simulink model "Proj2_P4_2"  (Simulink 8.6)
settings: Solver=ode45  StartTime=0.0  StopTime=10  MaxStep=0.001  RelTol=1e-3
values from neighbouring files (symbols this model uses):
  fl_rd_0 = fl_rd_rated    [Proj2_IM_IC_rated.m]    (also in Proj2_P1_calc.m = eps)
  fl_rd_0_est2 = fl_rd_rated_est2    [Proj2_P4_S2.m]    (also in Proj2_P4_calc2.m = fl_rd_0; Proj2_P4_calc3.m = fl_rd_0)
  fl_rd_0_est3 = fl_rd_rated    [Proj2_P4_S3.m]    (also in Proj2_P4_calc2.m = fl_rd_0; Proj2_P4_calc3.m = fl_rd_0)
  fl_sd_0 = fl_sd_rated    [Proj2_IM_IC_rated.m]    (also in Proj2_P1_calc.m = 0)
  fl_sq_0 = fl_sq_rated    [Proj2_IM_IC_rated.m]    (also in Proj2_P1_calc.m = 0)
  Isd_rated = real(Is_rated)    [Proj2_IM_IC_rated.m]
  Isd_rated_est2 = real(Is_rated_est2)    [Proj2_P4_S2.m]    (also in Proj2_P4_calc2.m = Isd_rated)
  Isd_rated_est3 = real(Is_rated_est3)    [Proj2_P4_S3.m]    (also in Proj2_P4_calc2.m = Isd_rated)
  Isq_0 = Isq_rated    [Proj2_IM_IC_rated.m]
  Isq_0_est2 = Isq_rated_est2    [Proj2_P4_S2.m]    (also in Proj2_P4_calc2.m = Isq_0; Proj2_P4_calc3.m = Isq_0)
  Isq_0_est3 = Isq_rated_est3    [Proj2_P4_S3.m]    (also in Proj2_P4_calc2.m = Isq_0; Proj2_P4_calc3.m = Isq_0)
  J_eq = 75    [Proj2_IM_parameters.m]
  Ki_i = w_c_i*sqrt(R_s^2+(w_c_i*L_s*sigma)^2) / sqrt(1+wc_Kp_by_Ki_for_i^2)    [Proj2_IM_IC_rated.m]
  Ki_i_est3 = w_c_i*sqrt(R_s^2+(w_c_i*L_s*sigma_est3)^2) / sqrt(1+wc_Kp_by_Ki_for_i_est3^2)    [Proj2_P4_S3.m]    (also in Proj2_P4_calc2.m = Ki_i)
  Ki_s = w_c_s^2*J_eq/(k*sqrt(1+tan(PM_s)^2))    [Proj2_IM_IC_rated.m]
  Ki_s_est2 = w_c_s^2*J_eq/(k_est2*sqrt(1+tan(PM_s)^2))    [Proj2_P4_S2.m]    (also in Proj2_P4_calc2.m = Ki_s)
  Ki_s_est3 = w_c_s^2*J_eq/(k_est3*sqrt(1+tan(PM_s)^2))    [Proj2_P4_S3.m]    (also in Proj2_P4_calc2.m = Ki_s)
  Kp_i = Ki_i * wc_Kp_by_Ki_for_i / w_c_i    [Proj2_IM_IC_rated.m]
  Kp_i_est3 = Ki_i_est3 * wc_Kp_by_Ki_for_i_est3 / w_c_i    [Proj2_P4_S3.m]    (also in Proj2_P4_calc2.m = Kp_i)
  Kp_s = Ki_s * wc_Kp_by_Ki_for_s / w_c_s    [Proj2_IM_IC_rated.m]
  Kp_s_est2 = Ki_s_est2 * wc_Kp_by_Ki_for_s / w_c_s    [Proj2_P4_S2.m]    (also in Proj2_P4_calc2.m = Kp_s)
  Kp_s_est3 = Ki_s_est3 * wc_Kp_by_Ki_for_s / w_c_s    [Proj2_P4_S3.m]    (also in Proj2_P4_calc2.m = Kp_s)
  L_m = X_m /w_syn    (= 0.00152788745368)    [Proj2_IM_parameters.m]
  L_r = L_lr+L_m    (= 0.00161011750761)    [Proj2_IM_parameters.m]
  L_r_est3 = L_lr_est3 + L_m    [Proj2_P4_S3.m]
  L_s = L_ls+L_m    (= 0.00161807525477)    [Proj2_IM_parameters.m]
  p = 6    [Proj2_IM_parameters.m]
  R_s = 1.4*10^-3    (= 0.0014)    [Proj2_IM_parameters.m]
  T_L_rated = T_em_rated    [Proj2_IM_parameters.m]
  tau_r = L_r/R_r    (= 1.62474016914)    [Proj2_IM_parameters.m]
  tau_r_est2 = L_r/R_r_est2    [Proj2_P4_S2.m]
  tau_r_est3 = L_r_est3/R_r    [Proj2_P4_S3.m]
  theta_da_0 = theta_fl_rated_a    [Proj2_IM_IC_rated.m]    (also in Proj2_P1_calc.m = 0)
  theta_dA_0 = theta_fl_rated_a    [Proj2_IM_IC_rated.m]    (also in Proj2_P1_calc.m = 0)
  theta_da_0_est2 = theta_fl_rated_a_est2    [Proj2_P4_S2.m]    (also in Proj2_P4_calc2.m = theta_da_0; Proj2_P4_calc3.m = theta_da_0)
  theta_da_0_est3 = theta_fl_rated_a_est3    [Proj2_P4_S3.m]    (also in Proj2_P4_calc2.m = theta_da_0; Proj2_P4_calc3.m = theta_da_0)
  Vsd_0 = Vsd_rated    [Proj2_IM_IC_rated.m]
  Vsd_prime_0 = Vsd_0 - L_m/L_r*d_fl_rd_0_by_dt + w_syn*sigma*L_s*Isq_0    [Proj2_IM_IC_rated.m]
  Vsq_0 = Vsq_rated    [Proj2_IM_IC_rated.m]
  Vsq_prime_0 = Vsq_0 - w_syn*(L_m/L_r)*fl_rd_0 - w_syn*sigma*L_s*Isd_0    [Proj2_IM_IC_rated.m]
  w_mech_0 = w_mech_rated    [Proj2_IM_IC_rated.m]    (also in Proj2_P1_calc.m = 0)
  w_mech_rated = (1-s)*w_syn/(p/2)    (= 124.407069082)    [Proj2_IM_parameters.m]
(part 1 of 2)
settings Model: Creator=XP  LastModifiedBy=XP
settings DataIOCC: SaveFormat=Dataset  SignalLoggingSaveFormat=Dataset
settings OptimizationCC: ExpressionDepthLimit=128
settings DebuggingCC: UnderspecifiedInitializationDetection=Simplified  MergeDetectMultiDrivingBlocksExec=error  SolverPrmCheckMsg=none  FcnCallInpInsideContextMsg=EnableAllAsError  StateNameClashWarn=none
settings HardwareCC: ProdBitPerPointer=64  ProdLargestAtomicFloat=Float  ProdIntDivRoundTo=Zero  ProdEndianess=LittleEndian  ProdWordSize=64  ProdHWDeviceType=Intel->x86-64 (Windows64)
settings GRTTargetCC: GeneratePreprocessorConditionals=Use local settings  CombineOutputUpdateFcns=on  GRTInterface=off
settings ConfigComp: CovModelRefEnable=off

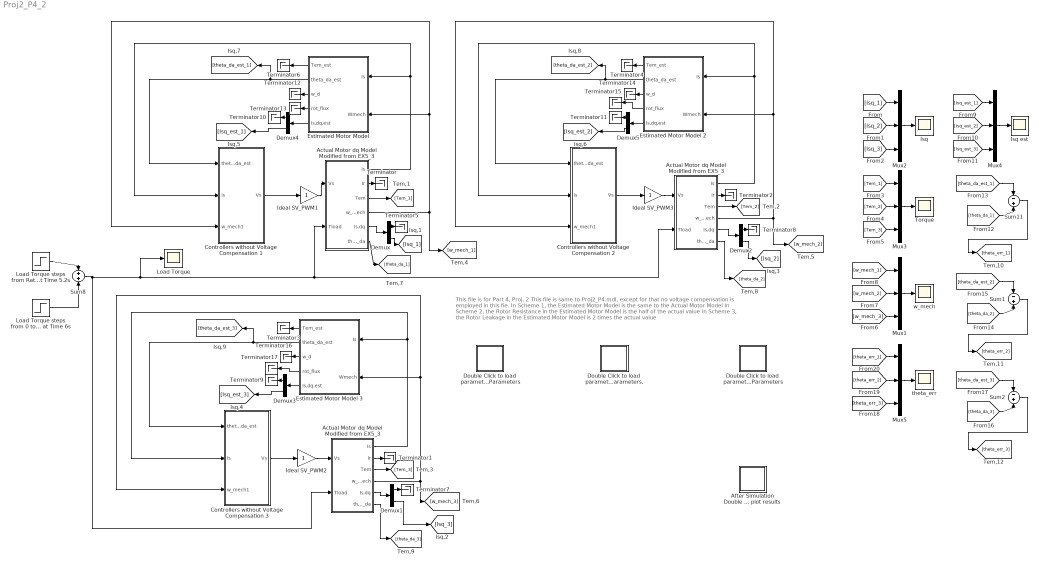
== system Proj2_P4_2 ==
  note: This file is for Part 4, Proj. 2
      | This file is same to Proj2_P4.mdl, except for that no voltage compensation is employed in this fie.
      |
      | In Scheme 1, the Estimated Motor Model is the same to the Actual Motor Model
      | In Scheme 2, the Rotor Resistance in the Estimated Motor Model is the half of the actual value
      | In Scheme 3, the Rotor Leakage in the Estimated Motor Model is 2 times the actual value
  Actual Motor dq Model Modified from EX5_3 : Subsystem
  "Actual Motor dq Model Modified from EX5_3 " : Subsystem
  "Actual Motor dq Model Modified from EX5_3  " : Subsystem
  "After Simulation Double Click to plot results " : Subsystem
      settings: OpenFcn=Proj2_P4_plots
      mask Display:
      | plot(0,0)
      | plot(100,100)
      | disp('Plot')
  Controllers without Voltage Compensation 1 : Subsystem
  Controllers without Voltage Compensation 2 : Subsystem
  Controllers without Voltage Compensation 3 : Subsystem
  Demux{,1..5} (6 alike) : Demux  Outputs=2
  "Double Click to load parameters and initial conditions  In this case, all initial values are obtained based on Actual Parameters;  parameters of Estimated Motor and Voltage Compensation Mode are based on Estimated Parameters;  paramters of  Controllers are based on Actual Parameters.  " : Subsystem
      settings: OpenFcn=Proj2_P4_calc2
      mask Display:
      | plot(0,0)
      | plot(100,100)
      | disp('Start')
  "Double Click to load parameters and initial conditions  In this case, all initial values are obtained based on Actual Parameters;  parameters of Estimated Motor and Voltage Compensation Model and Controllers are all based on Estimated Parameters  " : Subsystem
      settings: OpenFcn=Proj2_P4_calc3
      mask Display:
      | plot(0,0)
      | plot(100,100)
      | disp('Start')
  "Double Click to load parameters and initial conditions  In this case, all parameters and initial values in Estimated Motor, Voltage Compensation  and Controller Mode are based on Estimated Parameters" : Subsystem
      settings: OpenFcn=Proj2_P4_calc
      mask Display:
      | plot(0,0)
      | plot(100,100)
      | disp('Start')
  Estimated Motor Model : Subsystem
  Estimated Motor Model 2 : Subsystem
  Estimated Motor Model 3 : Subsystem
  Ideal SV_PWM1 : Gain  SaturateOnIntegerOverflow=on  OutDataTypeStr=Inherit: Same as input  ParamDataTypeStr=Inherit: Same as input
  Ideal SV_PWM2 : Gain  SaturateOnIntegerOverflow=on  OutDataTypeStr=Inherit: Same as input  ParamDataTypeStr=Inherit: Same as input
  Ideal SV_PWM3 : Gain  SaturateOnIntegerOverflow=on  OutDataTypeStr=Inherit: Same as input  ParamDataTypeStr=Inherit: Same as input
  Isq : Scope
  Isq est : Scope
  Load Torque : Scope
  Load Torque steps from 0 to 3/4Rated value at Time 6s : Step  Time=6  After=3/4*T_L_rated  SampleTime=0
  Load Torque steps from Rated to 0 at Time 5.2s : Step  Time=5.2  Before=T_L_rated  After=0  SampleTime=0
  Mux{1..5} (5 alike) : Mux  Inputs=3
  Sum1 : Sum  Inputs=-|+  SaturateOnIntegerOverflow=on  InputSameDT=on  OutDataTypeStr=Inherit: Same as first input
  Sum11 : Sum  Inputs=-|+  SaturateOnIntegerOverflow=on  InputSameDT=on  OutDataTypeStr=Inherit: Same as first input
  Sum2 : Sum  Inputs=-|+  SaturateOnIntegerOverflow=on  InputSameDT=on  OutDataTypeStr=Inherit: Same as first input
  Sum8 : Sum  SaturateOnIntegerOverflow=on  InputSameDT=on  OutDataTypeStr=Inherit: Same as first input
  Terminator{,1..17} (18 alike) : Terminator
  Torque : Scope
  theta_err : Scope
  w_mech : Scope
  wires:
  Actual Motor dq Model Modified from EX5_3/2(Ir) -> Terminator/1
  Ideal SV_PWM1/1 -> Actual Motor dq Model Modified from EX5_3/1(Vs)
  Actual Motor dq Model Modified from EX5_3/1(Is) -> Controllers without Voltage Compensation 1/2(Is), Estimated Motor Model/1(Is)
  Controllers without Voltage Compensation 1/1(Vs) -> Ideal SV_PWM1/1
  Estimated Motor Model/2(theta_da_est) -> [theta_da_est_1], Controllers without Voltage Compensation 1/1(theta_da_est)
  Actual Motor dq Model Modified from EX5_3/4(w_mech) -> [w_mech_1], Controllers without Voltage Compensation 1/3(w_mech1), Estimated Motor Model/2(Wmech)
  "Actual Motor dq Model Modified from EX5_3  "/2(Ir) -> Terminator1/1
  Ideal SV_PWM2/1 -> "Actual Motor dq Model Modified from EX5_3  "/1(Vs)
  "Actual Motor dq Model Modified from EX5_3  "/1(Is) -> Controllers without Voltage Compensation 3/2(Is), Estimated Motor Model 3/1(Is)
  Estimated Motor Model 3/2(theta_da_est) -> [theta_da_est_3], Controllers without Voltage Compensation 3/1(theta_da_est)
  "Actual Motor dq Model Modified from EX5_3  "/4(w_mech) -> [w_mech_3], Controllers without Voltage Compensation 3/3(w_mech1), Estimated Motor Model 3/2(Wmech)
  "Actual Motor dq Model Modified from EX5_3 "/2(Ir) -> Terminator2/1
  Ideal SV_PWM3/1 -> "Actual Motor dq Model Modified from EX5_3 "/1(Vs)
  Sum8/1 -> "Actual Motor dq Model Modified from EX5_3  "/2(Tload), "Actual Motor dq Model Modified from EX5_3 "/2(Tload), Actual Motor dq Model Modified from EX5_3/2(Tload), Load Torque/1
  "Actual Motor dq Model Modified from EX5_3 "/1(Is) -> Estimated Motor Model 2/1(Is), Controllers without Voltage Compensation 2/2(Is)
  Estimated Motor Model 2/2(theta_da_est) -> [theta_da_est_2], Controllers without Voltage Compensation 2/1(theta_da_est)
  "Actual Motor dq Model Modified from EX5_3 "/4(w_mech) -> [w_mech_2], Controllers without Voltage Compensation 2/3(w_mech1), Estimated Motor Model 2/2(Wmech)
  Controllers without Voltage Compensation 3/1(Vs) -> Ideal SV_PWM2/1
  Controllers without Voltage Compensation 2/1(Vs) -> Ideal SV_PWM3/1
  Estimated Motor Model/1(Tem_est) -> Terminator6/1
  Estimated Motor Model 3/1(Tem_est) -> Terminator3/1
  Estimated Motor Model 2/1(Tem_est) -> Terminator4/1
  Actual Motor dq Model Modified from EX5_3/5(Is,dq) -> Demux/1
  Demux/1 -> Terminator5/1
  "Actual Motor dq Model Modified from EX5_3  "/5(Is,dq) -> Demux1/1
  Demux1/1 -> Terminator7/1
  "Actual Motor dq Model Modified from EX5_3 "/5(Is,dq) -> Demux2/1
  Demux2/1 -> Terminator8/1
  Demux/2 -> [Isq_1]
  Demux1/2 -> [Isq_3]
  Demux2/2 -> [Isq_2]
  Actual Motor dq Model Modified from EX5_3/3(Tem) -> [Tem_1]
  "Actual Motor dq Model Modified from EX5_3 "/3(Tem) -> [Tem_2]
  "Actual Motor dq Model Modified from EX5_3  "/3(Tem) -> [Tem_3]
  Estimated Motor Model 3/5(Is,dq,est) -> Demux3/1
  Demux3/1 -> Terminator9/1
  Demux3/2 -> [Isq_est_3]
  Estimated Motor Model/5(Is,dq,est) -> Demux4/1
  Demux4/1 -> Terminator10/1
  Demux4/2 -> [Isq_est_1]
  Estimated Motor Model 2/5(Is,dq,est) -> Demux5/1
  Demux5/1 -> Terminator11/1
  Demux5/2 -> [Isq_est_2]
  Actual Motor dq Model Modified from EX5_3/6(theta_da) -> [theta_da_1]
  "Actual Motor dq Model Modified from EX5_3 "/6(theta_da) -> [theta_da_2]
  "Actual Motor dq Model Modified from EX5_3  "/6(theta_da) -> [theta_da_3]
  Load Torque steps from Rated to 0 at Time 5.2s/1 -> Sum8/1
  Load Torque steps from 0 to 3/4Rated value at Time 6s/1 -> Sum8/2
  [theta_err_1] -> Mux5/1
  Mux3/1 -> Torque/1
  Mux1/1 -> w_mech/1
  [Tem_2] -> Mux3/2
  [Tem_3] -> Mux3/3
  [w_mech_3] -> Mux1/3
  [w_mech_2] -> Mux1/2
  [w_mech_1] -> Mux1/1
  [Isq_1] -> Mux2/1
  [Isq_2] -> Mux2/2
  [Isq_3] -> Mux2/3
  Mux2/1 -> Isq/1
  [Tem_1] -> Mux3/1
  [Isq_est_1] -> Mux4/1
  [Isq_est_2] -> Mux4/2
  [Isq_est_3] -> Mux4/3
  Mux4/1 -> Isq est/1
  [theta_da_est_1] -> Sum11/1
  [theta_da_1] -> Sum11/2
  [theta_da_est_2] -> Sum1/1
  [theta_da_2] -> Sum1/2
  [theta_da_est_3] -> Sum2/1
  [theta_da_3] -> Sum2/2
  Sum11/1 -> [theta_err_1]
  Sum1/1 -> [theta_err_2]
  Sum2/1 -> [theta_err_3]
  Mux5/1 -> theta_err/1
  [theta_err_3] -> Mux5/3
  [theta_err_2] -> Mux5/2
  Estimated Motor Model/3(w_d) -> Terminator12/1
  Estimated Motor Model/4(rot_flux) -> Terminator13/1
  Estimated Motor Model 2/3(w_d) -> Terminator14/1
  Estimated Motor Model 2/4(rot_flux) -> Terminator15/1
  Estimated Motor Model 3/3(w_d) -> Terminator16/1
  Estimated Motor Model 3/4(rot_flux) -> Terminator17/1

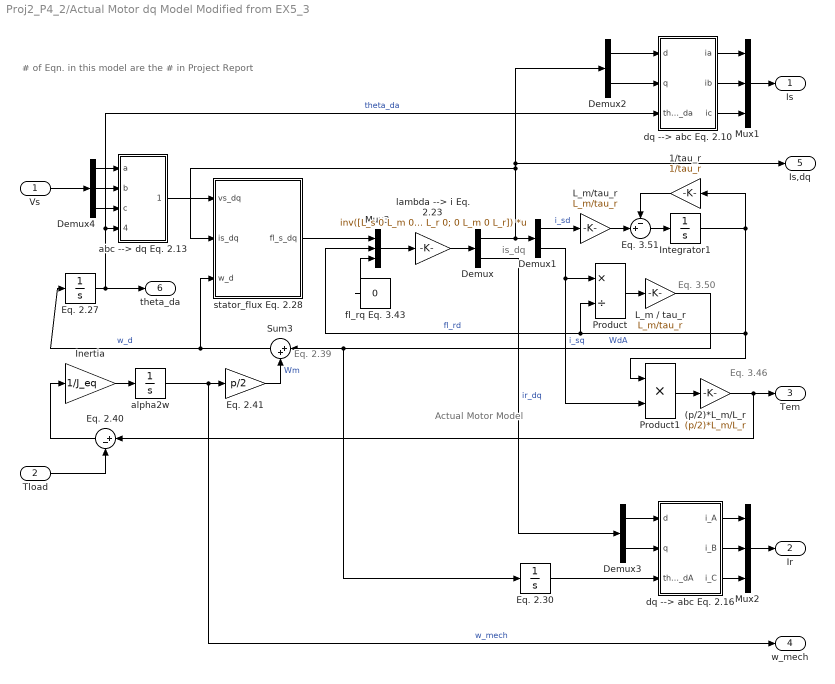
== system Proj2_P4_2/Actual Motor dq Model Modified from EX5_3 ==
  note: Eq. 2.39
  note: Eq. 3.46
  note: Eq. 3.50
  note: # of Eqn. in this model are the # in Project Report
  note: Actual Motor Model
  note: is_dq
  Vs : Inport
  Tload : Inport  Port=2
  (p/2)*L_m/L_r : Gain  Gain=(p/2)*L_m/L_r  SaturateOnIntegerOverflow=on  OutDataTypeStr=Inherit: Same as input  ParamDataTypeStr=Inherit: Same as input
  1/tau_r : Gain  Gain=1/tau_r  SaturateOnIntegerOverflow=on  OutDataTypeStr=Inherit: Same as input  ParamDataTypeStr=Inherit: Same as input
  Demux{,1..3} (4 alike) : Demux  Outputs=2
  Demux4 : Demux  Outputs=3
  Eq. 2.27 : Integrator  InitialCondition=theta_da_0
  Eq. 2.30 : Integrator  InitialCondition=theta_dA_0
  Eq. 2.40 : Sum  Inputs=|+-  SaturateOnIntegerOverflow=on  InputSameDT=on  OutDataTypeStr=Inherit: Same as first input
  Eq. 2.41 : Gain  Gain=p/2  SaturateOnIntegerOverflow=on  OutDataTypeStr=Inherit: Same as input  ParamDataTypeStr=Inherit: Same as input
  Eq. 3.51 : Sum  Inputs=-+|  SaturateOnIntegerOverflow=on  InputSameDT=on  OutDataTypeStr=Inherit: Same as first input
  Inertia : Gain  Gain=1/J_eq  SaturateOnIntegerOverflow=on  OutDataTypeStr=Inherit: Same as input  ParamDataTypeStr=Inherit: Same as input
  Integrator1 : Integrator  InitialCondition=fl_rd_0
  L_m / tau_r : Gain  Gain=L_m/tau_r  SaturateOnIntegerOverflow=on  OutDataTypeStr=Inherit: Same as input  ParamDataTypeStr=Inherit: Same as input
  L_m/tau_r : Gain  Gain=L_m/tau_r  SaturateOnIntegerOverflow=on  OutDataTypeStr=Inherit: Same as input  ParamDataTypeStr=Inherit: Same as input
  Mux1 : Mux  Inputs=3
  Mux2 : Mux  Inputs=3
  Mux3 : Mux  Inputs=3
  Product : Product  Inputs=*/  SaturateOnIntegerOverflow=on  RndMeth=Zero  InputSameDT=on  OutDataTypeStr=Inherit: Same as first input
  Product1 : Product  SaturateOnIntegerOverflow=on  RndMeth=Zero  InputSameDT=on  OutDataTypeStr=Inherit: Same as first input
  Sum3 : Sum  Inputs=|++  SaturateOnIntegerOverflow=on  InputSameDT=on  OutDataTypeStr=Inherit: Same as first input
  abc --> dq Eq. 2.13 : Subsystem
  alpha2w : Integrator  InitialCondition=w_mech_0
  dq --> abc Eq. 2.10 : Subsystem
  "dq --> abc Eq. 2.16 " : Subsystem
  fl_rq Eq. 3.43 : Constant  Value=0
  lambda --> i Eq. 2.23 : Gain  Gain=inv([L_s 0 L_m 0; 0 L_s 0 L_m; L_m 0 L_r 0; 0 L_m 0 L_r])  Multiplication=Matrix(K*u)  SaturateOnIntegerOverflow=on  OutDataTypeStr=Inherit: Same as input  ParamDataTypeStr=Inherit: Same as input
  stator_flux Eq. 2.28 : Subsystem
  Is : Outport
  Ir : Outport  Port=2
  Tem : Outport  Port=3
  w_mech : Outport  Port=4
  Is,dq : Outport  Port=5
  theta_da : Outport  Port=6
  wires:
  Mux3/1 -> lambda --> i Eq. 2.23/1
  Demux/1 -> Demux1/1, Is,dq/1, Demux2/1, stator_flux Eq. 2.28/2(is_dq)
  Eq. 2.27/1 -> theta_da/1, dq --> abc Eq. 2.10/3(theta_da), abc --> dq Eq. 2.13/4(theta_da)  "theta_da"
  stator_flux Eq. 2.28/1(fl_s_dq) -> Mux3/1
  abc --> dq Eq. 2.13/1(vs_dq) -> stator_flux Eq. 2.28/1(vs_dq)
  lambda --> i Eq. 2.23/1 -> Demux/1
  Demux1/1 -> L_m/tau_r/1  "i_sd"
  L_m/tau_r/1 -> Eq. 3.51/2
  1/tau_r/1 -> Eq. 3.51/1
  Eq. 3.51/1 -> Integrator1/1
  Demux1/2 -> Product/1, Product1/2  "i_sq"
  Product/1 -> L_m / tau_r/1
  L_m / tau_r/1 -> Sum3/1, Eq. 2.30/1  "WdA"
  Product1/1 -> (p/2)*L_m/L_r/1
  fl_rq Eq. 3.43/1 -> Mux3/3
  Sum3/1 -> Eq. 2.27/1, stator_flux Eq. 2.28/3(w_d)  "w_d"
  (p/2)*L_m/L_r/1 -> Tem/1, Eq. 2.40/1
  Demux2/1 -> dq --> abc Eq. 2.10/1(d)
  Demux2/2 -> dq --> abc Eq. 2.10/2(q)
  dq --> abc Eq. 2.10/1(ia) -> Mux1/1
  dq --> abc Eq. 2.10/2(ib) -> Mux1/2
  dq --> abc Eq. 2.10/3(ic) -> Mux1/3
  Integrator1/1 -> 1/tau_r/1, Mux3/2, Product/2, Product1/1  "fl_rd"
  Eq. 2.41/1 -> Sum3/2  "Wm"
  Demux/2 -> Demux3/1  "ir_dq"
  Eq. 2.40/1 -> Inertia/1
  Inertia/1 -> alpha2w/1
  alpha2w/1 -> w_mech/1, Eq. 2.41/1  "w_mech"
  Tload/1 -> Eq. 2.40/2
  Mux1/1 -> Is/1
  Demux3/1 -> "dq --> abc Eq. 2.16 "/1(d)
  Demux3/2 -> "dq --> abc Eq. 2.16 "/2(q)
  Eq. 2.30/1 -> "dq --> abc Eq. 2.16 "/3(theta_dA)
  "dq --> abc Eq. 2.16 "/1(i_A) -> Mux2/1
  "dq --> abc Eq. 2.16 "/2(i_B) -> Mux2/2
  "dq --> abc Eq. 2.16 "/3(i_C) -> Mux2/3
  Mux2/1 -> Ir/1
  Demux4/1 -> abc --> dq Eq. 2.13/1(a)
  Demux4/2 -> abc --> dq Eq. 2.13/2(b)
  Demux4/3 -> abc --> dq Eq. 2.13/3(c)
  Vs/1 -> Demux4/1

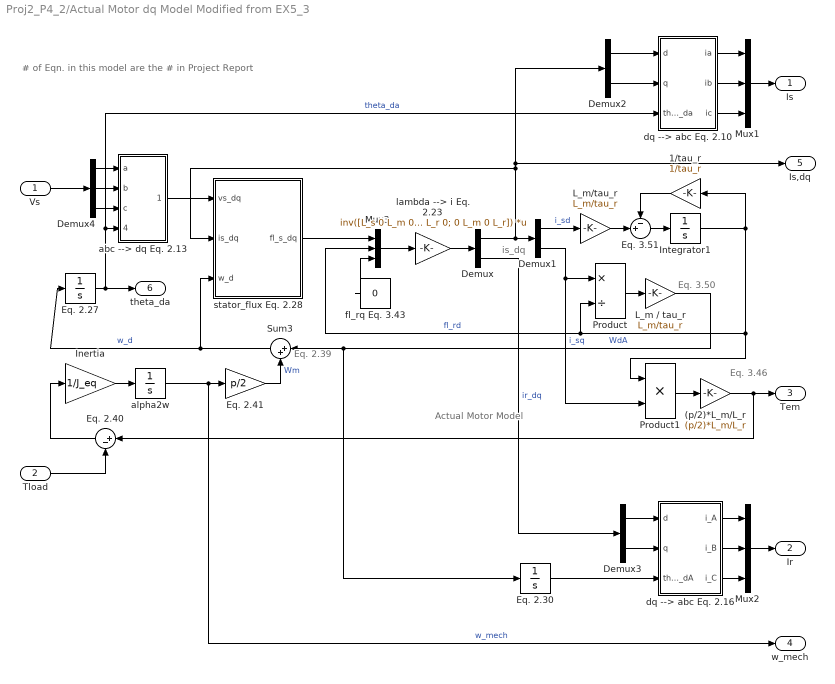
== system Proj2_P4_2/Actual Motor dq Model Modified from EX5_3  ==
  note: Eq. 2.39
  note: Eq. 3.46
  note: Eq. 3.50
  note: # of Eqn. in this model are the # in Project Report
  note: Actual Motor Model
  note: is_dq
  Vs : Inport
  Tload : Inport  Port=2
  (p/2)*L_m/L_r : Gain  Gain=(p/2)*L_m/L_r  SaturateOnIntegerOverflow=on  OutDataTypeStr=Inherit: Same as input  ParamDataTypeStr=Inherit: Same as input
  1/tau_r : Gain  Gain=1/tau_r  SaturateOnIntegerOverflow=on  OutDataTypeStr=Inherit: Same as input  ParamDataTypeStr=Inherit: Same as input
  Demux{,1..3} (4 alike) : Demux  Outputs=2
  Demux4 : Demux  Outputs=3
  Eq. 2.27 : Integrator  InitialCondition=theta_da_0
  Eq. 2.30 : Integrator  InitialCondition=theta_dA_0
  Eq. 2.40 : Sum  Inputs=|+-  SaturateOnIntegerOverflow=on  InputSameDT=on  OutDataTypeStr=Inherit: Same as first input
  Eq. 2.41 : Gain  Gain=p/2  SaturateOnIntegerOverflow=on  OutDataTypeStr=Inherit: Same as input  ParamDataTypeStr=Inherit: Same as input
  Eq. 3.51 : Sum  Inputs=-+|  SaturateOnIntegerOverflow=on  InputSameDT=on  OutDataTypeStr=Inherit: Same as first input
  Inertia : Gain  Gain=1/J_eq  SaturateOnIntegerOverflow=on  OutDataTypeStr=Inherit: Same as input  ParamDataTypeStr=Inherit: Same as input
  Integrator1 : Integrator  InitialCondition=fl_rd_0
  L_m / tau_r : Gain  Gain=L_m/tau_r  SaturateOnIntegerOverflow=on  OutDataTypeStr=Inherit: Same as input  ParamDataTypeStr=Inherit: Same as input
  L_m/tau_r : Gain  Gain=L_m/tau_r  SaturateOnIntegerOverflow=on  OutDataTypeStr=Inherit: Same as input  ParamDataTypeStr=Inherit: Same as input
  Mux1 : Mux  Inputs=3
  Mux2 : Mux  Inputs=3
  Mux3 : Mux  Inputs=3
  Product : Product  Inputs=*/  SaturateOnIntegerOverflow=on  RndMeth=Zero  InputSameDT=on  OutDataTypeStr=Inherit: Same as first input
  Product1 : Product  SaturateOnIntegerOverflow=on  RndMeth=Zero  InputSameDT=on  OutDataTypeStr=Inherit: Same as first input
  Sum3 : Sum  Inputs=|++  SaturateOnIntegerOverflow=on  InputSameDT=on  OutDataTypeStr=Inherit: Same as first input
  abc --> dq Eq. 2.13 : Subsystem
  alpha2w : Integrator  InitialCondition=w_mech_0
  dq --> abc Eq. 2.10 : Subsystem
  "dq --> abc Eq. 2.16 " : Subsystem
  fl_rq Eq. 3.43 : Constant  Value=0
  lambda --> i Eq. 2.23 : Gain  Gain=inv([L_s 0 L_m 0; 0 L_s 0 L_m; L_m 0 L_r 0; 0 L_m 0 L_r])  Multiplication=Matrix(K*u)  SaturateOnIntegerOverflow=on  OutDataTypeStr=Inherit: Same as input  ParamDataTypeStr=Inherit: Same as input
  stator_flux Eq. 2.28 : Subsystem
  Is : Outport
  Ir : Outport  Port=2
  Tem : Outport  Port=3
  w_mech : Outport  Port=4
  Is,dq : Outport  Port=5
  theta_da : Outport  Port=6
  wires:
  Mux3/1 -> lambda --> i Eq. 2.23/1
  Demux/1 -> Demux1/1, Is,dq/1, Demux2/1, stator_flux Eq. 2.28/2(is_dq)
  Eq. 2.27/1 -> theta_da/1, dq --> abc Eq. 2.10/3(theta_da), abc --> dq Eq. 2.13/4(theta_da)  "theta_da"
  stator_flux Eq. 2.28/1(fl_s_dq) -> Mux3/1
  abc --> dq Eq. 2.13/1(vs_dq) -> stator_flux Eq. 2.28/1(vs_dq)
  lambda --> i Eq. 2.23/1 -> Demux/1
  Demux1/1 -> L_m/tau_r/1  "i_sd"
  L_m/tau_r/1 -> Eq. 3.51/2
  1/tau_r/1 -> Eq. 3.51/1
  Eq. 3.51/1 -> Integrator1/1
  Demux1/2 -> Product/1, Product1/2  "i_sq"
  Product/1 -> L_m / tau_r/1
  L_m / tau_r/1 -> Sum3/1, Eq. 2.30/1  "WdA"
  Product1/1 -> (p/2)*L_m/L_r/1
  fl_rq Eq. 3.43/1 -> Mux3/3
  Sum3/1 -> Eq. 2.27/1, stator_flux Eq. 2.28/3(w_d)  "w_d"
  (p/2)*L_m/L_r/1 -> Tem/1, Eq. 2.40/1
  Demux2/1 -> dq --> abc Eq. 2.10/1(d)
  Demux2/2 -> dq --> abc Eq. 2.10/2(q)
  dq --> abc Eq. 2.10/1(ia) -> Mux1/1
  dq --> abc Eq. 2.10/2(ib) -> Mux1/2
  dq --> abc Eq. 2.10/3(ic) -> Mux1/3
  Integrator1/1 -> 1/tau_r/1, Mux3/2, Product/2, Product1/1  "fl_rd"
  Eq. 2.41/1 -> Sum3/2  "Wm"
  Demux/2 -> Demux3/1  "ir_dq"
  Eq. 2.40/1 -> Inertia/1
  Inertia/1 -> alpha2w/1
  alpha2w/1 -> w_mech/1, Eq. 2.41/1  "w_mech"
  Tload/1 -> Eq. 2.40/2
  Mux1/1 -> Is/1
  Demux3/1 -> "dq --> abc Eq. 2.16 "/1(d)
  Demux3/2 -> "dq --> abc Eq. 2.16 "/2(q)
  Eq. 2.30/1 -> "dq --> abc Eq. 2.16 "/3(theta_dA)
  "dq --> abc Eq. 2.16 "/1(i_A) -> Mux2/1
  "dq --> abc Eq. 2.16 "/2(i_B) -> Mux2/2
  "dq --> abc Eq. 2.16 "/3(i_C) -> Mux2/3
  Mux2/1 -> Ir/1
  Demux4/1 -> abc --> dq Eq. 2.13/1(a)
  Demux4/2 -> abc --> dq Eq. 2.13/2(b)
  Demux4/3 -> abc --> dq Eq. 2.13/3(c)
  Vs/1 -> Demux4/1

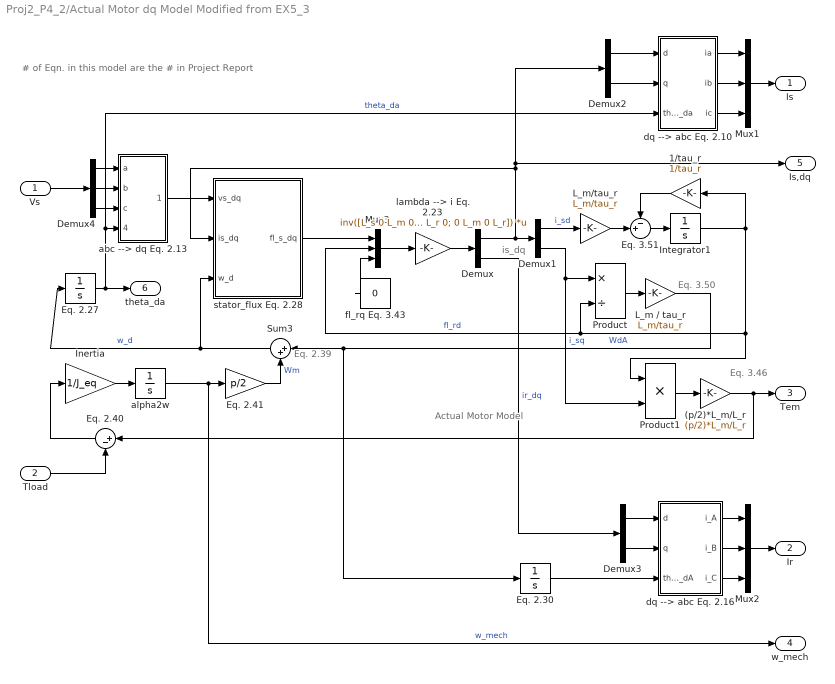
== system Proj2_P4_2/Actual Motor dq Model Modified from EX5_3   ==
  note: Eq. 2.39
  note: Eq. 3.46
  note: Eq. 3.50
  note: # of Eqn. in this model are the # in Project Report
  note: Actual Motor Model
  note: is_dq
  Vs : Inport
  Tload : Inport  Port=2
  (p/2)*L_m/L_r : Gain  Gain=(p/2)*L_m/L_r  SaturateOnIntegerOverflow=on  OutDataTypeStr=Inherit: Same as input  ParamDataTypeStr=Inherit: Same as input
  1/tau_r : Gain  Gain=1/tau_r  SaturateOnIntegerOverflow=on  OutDataTypeStr=Inherit: Same as input  ParamDataTypeStr=Inherit: Same as input
  Demux{,1..3} (4 alike) : Demux  Outputs=2
  Demux4 : Demux  Outputs=3
  Eq. 2.27 : Integrator  InitialCondition=theta_da_0
  Eq. 2.30 : Integrator  InitialCondition=theta_dA_0
  Eq. 2.40 : Sum  Inputs=|+-  SaturateOnIntegerOverflow=on  InputSameDT=on  OutDataTypeStr=Inherit: Same as first input
  Eq. 2.41 : Gain  Gain=p/2  SaturateOnIntegerOverflow=on  OutDataTypeStr=Inherit: Same as input  ParamDataTypeStr=Inherit: Same as input
  Eq. 3.51 : Sum  Inputs=-+|  SaturateOnIntegerOverflow=on  InputSameDT=on  OutDataTypeStr=Inherit: Same as first input
  Inertia : Gain  Gain=1/J_eq  SaturateOnIntegerOverflow=on  OutDataTypeStr=Inherit: Same as input  ParamDataTypeStr=Inherit: Same as input
  Integrator1 : Integrator  InitialCondition=fl_rd_0
  L_m / tau_r : Gain  Gain=L_m/tau_r  SaturateOnIntegerOverflow=on  OutDataTypeStr=Inherit: Same as input  ParamDataTypeStr=Inherit: Same as input
  L_m/tau_r : Gain  Gain=L_m/tau_r  SaturateOnIntegerOverflow=on  OutDataTypeStr=Inherit: Same as input  ParamDataTypeStr=Inherit: Same as input
  Mux1 : Mux  Inputs=3
  Mux2 : Mux  Inputs=3
  Mux3 : Mux  Inputs=3
  Product : Product  Inputs=*/  SaturateOnIntegerOverflow=on  RndMeth=Zero  InputSameDT=on  OutDataTypeStr=Inherit: Same as first input
  Product1 : Product  SaturateOnIntegerOverflow=on  RndMeth=Zero  InputSameDT=on  OutDataTypeStr=Inherit: Same as first input
  Sum3 : Sum  Inputs=|++  SaturateOnIntegerOverflow=on  InputSameDT=on  OutDataTypeStr=Inherit: Same as first input
  abc --> dq Eq. 2.13 : Subsystem
  alpha2w : Integrator  InitialCondition=w_mech_0
  dq --> abc Eq. 2.10 : Subsystem
  "dq --> abc Eq. 2.16 " : Subsystem
  fl_rq Eq. 3.43 : Constant  Value=0
  lambda --> i Eq. 2.23 : Gain  Gain=inv([L_s 0 L_m 0; 0 L_s 0 L_m; L_m 0 L_r 0; 0 L_m 0 L_r])  Multiplication=Matrix(K*u)  SaturateOnIntegerOverflow=on  OutDataTypeStr=Inherit: Same as input  ParamDataTypeStr=Inherit: Same as input
  stator_flux Eq. 2.28 : Subsystem
  Is : Outport
  Ir : Outport  Port=2
  Tem : Outport  Port=3
  w_mech : Outport  Port=4
  Is,dq : Outport  Port=5
  theta_da : Outport  Port=6
  wires:
  Mux3/1 -> lambda --> i Eq. 2.23/1
  Demux/1 -> Demux1/1, Is,dq/1, Demux2/1, stator_flux Eq. 2.28/2(is_dq)
  Eq. 2.27/1 -> theta_da/1, dq --> abc Eq. 2.10/3(theta_da), abc --> dq Eq. 2.13/4(theta_da)  "theta_da"
  stator_flux Eq. 2.28/1(fl_s_dq) -> Mux3/1
  abc --> dq Eq. 2.13/1(vs_dq) -> stator_flux Eq. 2.28/1(vs_dq)
  lambda --> i Eq. 2.23/1 -> Demux/1
  Demux1/1 -> L_m/tau_r/1  "i_sd"
  L_m/tau_r/1 -> Eq. 3.51/2
  1/tau_r/1 -> Eq. 3.51/1
  Eq. 3.51/1 -> Integrator1/1
  Demux1/2 -> Product/1, Product1/2  "i_sq"
  Product/1 -> L_m / tau_r/1
  L_m / tau_r/1 -> Sum3/1, Eq. 2.30/1  "WdA"
  Product1/1 -> (p/2)*L_m/L_r/1
  fl_rq Eq. 3.43/1 -> Mux3/3
  Sum3/1 -> Eq. 2.27/1, stator_flux Eq. 2.28/3(w_d)  "w_d"
  (p/2)*L_m/L_r/1 -> Tem/1, Eq. 2.40/1
  Demux2/1 -> dq --> abc Eq. 2.10/1(d)
  Demux2/2 -> dq --> abc Eq. 2.10/2(q)
  dq --> abc Eq. 2.10/1(ia) -> Mux1/1
  dq --> abc Eq. 2.10/2(ib) -> Mux1/2
  dq --> abc Eq. 2.10/3(ic) -> Mux1/3
  Integrator1/1 -> 1/tau_r/1, Mux3/2, Product/2, Product1/1  "fl_rd"
  Eq. 2.41/1 -> Sum3/2  "Wm"
  Demux/2 -> Demux3/1  "ir_dq"
  Eq. 2.40/1 -> Inertia/1
  Inertia/1 -> alpha2w/1
  alpha2w/1 -> w_mech/1, Eq. 2.41/1  "w_mech"
  Tload/1 -> Eq. 2.40/2
  Mux1/1 -> Is/1
  Demux3/1 -> "dq --> abc Eq. 2.16 "/1(d)
  Demux3/2 -> "dq --> abc Eq. 2.16 "/2(q)
  Eq. 2.30/1 -> "dq --> abc Eq. 2.16 "/3(theta_dA)
  "dq --> abc Eq. 2.16 "/1(i_A) -> Mux2/1
  "dq --> abc Eq. 2.16 "/2(i_B) -> Mux2/2
  "dq --> abc Eq. 2.16 "/3(i_C) -> Mux2/3
  Mux2/1 -> Ir/1
  Demux4/1 -> abc --> dq Eq. 2.13/1(a)
  Demux4/2 -> abc --> dq Eq. 2.13/2(b)
  Demux4/3 -> abc --> dq Eq. 2.13/3(c)
  Vs/1 -> Demux4/1

== system Proj2_P4_2/After Simulation Double Click to plot results  ==

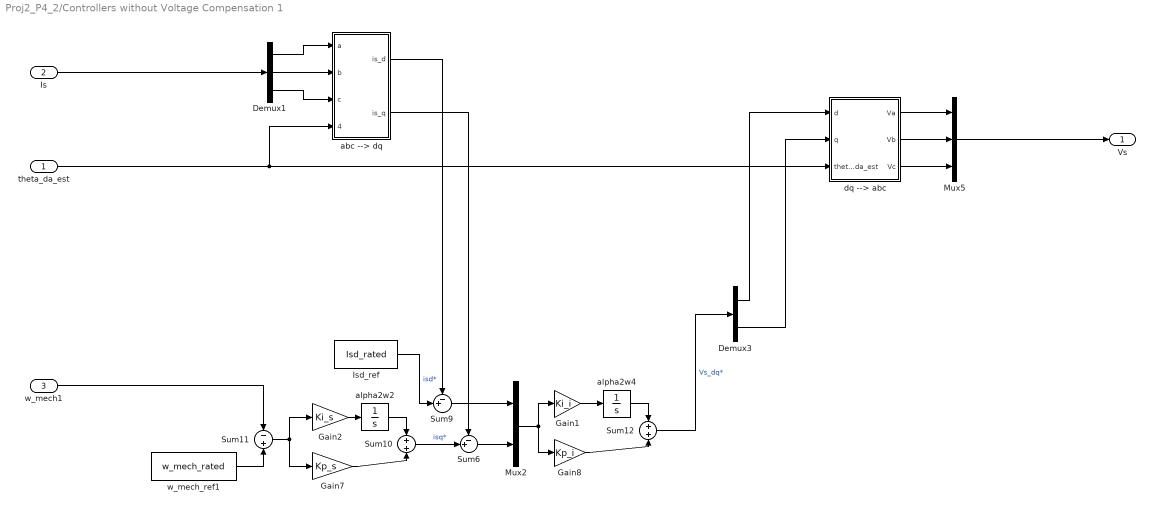
== system Proj2_P4_2/Controllers without Voltage Compensation 1 ==
  theta_da_est : Inport
  Is : Inport  Port=2
  w_mech1 : Inport  Port=3
  Demux1 : Demux  Outputs=3
  Demux3 : Demux  Outputs=2
  Gain1 : Gain  Gain=Ki_i  SaturateOnIntegerOverflow=on  OutDataTypeStr=Inherit: Same as input  ParamDataTypeStr=Inherit: Same as input
  Gain2 : Gain  Gain=Ki_s  SaturateOnIntegerOverflow=on  OutDataTypeStr=Inherit: Same as input  ParamDataTypeStr=Inherit: Same as input
  Gain7 : Gain  Gain=Kp_s  SaturateOnIntegerOverflow=on  OutDataTypeStr=Inherit: Same as input  ParamDataTypeStr=Inherit: Same as input
  Gain8 : Gain  Gain=Kp_i  SaturateOnIntegerOverflow=on  OutDataTypeStr=Inherit: Same as input  ParamDataTypeStr=Inherit: Same as input
  Isd_ref : Constant  Value=Isd_rated
  Mux2 : Mux  Inputs=2
  Mux5 : Mux  Inputs=3
  Sum10 : Sum  SaturateOnIntegerOverflow=on  InputSameDT=on  OutDataTypeStr=Inherit: Same as first input
  Sum11 : Sum  Inputs=-|+  SaturateOnIntegerOverflow=on  InputSameDT=on  OutDataTypeStr=Inherit: Same as first input
  Sum12 : Sum  SaturateOnIntegerOverflow=on  InputSameDT=on  OutDataTypeStr=Inherit: Same as first input
  Sum6 : Sum  Inputs=-+|  SaturateOnIntegerOverflow=on  InputSameDT=on  OutDataTypeStr=Inherit: Same as first input
  Sum9 : Sum  Inputs=-+|  SaturateOnIntegerOverflow=on  InputSameDT=on  OutDataTypeStr=Inherit: Same as first input
  abc --> dq : Subsystem
  alpha2w2 : Integrator  InitialCondition=Isq_0
  alpha2w4 : Integrator  InitialCondition=[Vsd_prime_0; Vsq_prime_0]
  "dq --> abc " : Subsystem
  w_mech_ref1 : Constant  Value=w_mech_rated
  Vs : Outport
  wires:
  Sum12/1 -> Demux3/1  "Vs_dq*"
  Demux1/2 -> abc --> dq/2(b)
  Demux1/1 -> abc --> dq/1(a)
  Demux1/3 -> abc --> dq/3(c)
  Is/1 -> Demux1/1
  "dq --> abc "/3(Vc) -> Mux5/3
  Sum6/1 -> Mux2/2
  abc --> dq/2(is_q) -> Sum6/1
  Demux3/1 -> "dq --> abc "/1(d)
  Sum10/1 -> Sum6/2  "isq*"
  Demux3/2 -> "dq --> abc "/2(q)
  Isd_ref/1 -> Sum9/2  "isd*"
  theta_da_est/1 -> abc --> dq/4(theta_da_est), "dq --> abc "/3(theta_da_est)
  alpha2w2/1 -> Sum10/1
  w_mech_ref1/1 -> Sum11/2
  w_mech1/1 -> Sum11/1
  "dq --> abc "/2(Vb) -> Mux5/2
  Gain2/1 -> alpha2w2/1
  abc --> dq/1(is_d) -> Sum9/1
  Mux5/1 -> Vs/1
  "dq --> abc "/1(Va) -> Mux5/1
  Mux2/1 -> Gain1/1, Gain8/1
  Gain1/1 -> alpha2w4/1
  Gain8/1 -> Sum12/2
  alpha2w4/1 -> Sum12/1
  Sum9/1 -> Mux2/1
  Gain7/1 -> Sum10/2
  Sum11/1 -> Gain2/1, Gain7/1

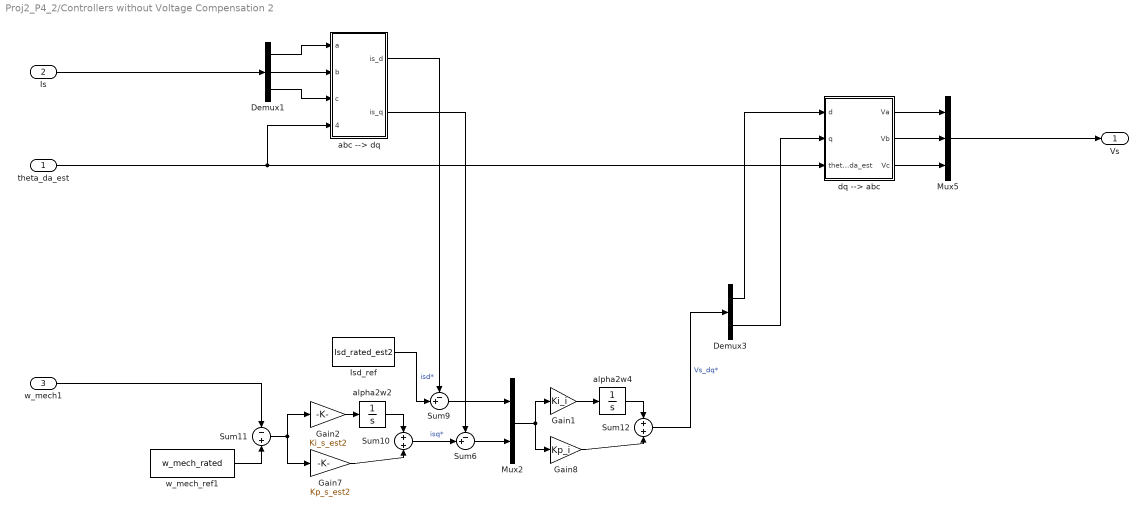
== system Proj2_P4_2/Controllers without Voltage Compensation 2 ==
  theta_da_est : Inport
  Is : Inport  Port=2
  w_mech1 : Inport  Port=3
  Demux1 : Demux  Outputs=3
  Demux3 : Demux  Outputs=2
  Gain1 : Gain  Gain=Ki_i  SaturateOnIntegerOverflow=on  OutDataTypeStr=Inherit: Same as input  ParamDataTypeStr=Inherit: Same as input
  Gain2 : Gain  Gain=Ki_s_est2  SaturateOnIntegerOverflow=on  OutDataTypeStr=Inherit: Same as input  ParamDataTypeStr=Inherit: Same as input
  Gain7 : Gain  Gain=Kp_s_est2  SaturateOnIntegerOverflow=on  OutDataTypeStr=Inherit: Same as input  ParamDataTypeStr=Inherit: Same as input
  Gain8 : Gain  Gain=Kp_i  SaturateOnIntegerOverflow=on  OutDataTypeStr=Inherit: Same as input  ParamDataTypeStr=Inherit: Same as input
  Isd_ref : Constant  Value=Isd_rated_est2
  Mux2 : Mux  Inputs=2
  Mux5 : Mux  Inputs=3
  Sum10 : Sum  SaturateOnIntegerOverflow=on  InputSameDT=on  OutDataTypeStr=Inherit: Same as first input
  Sum11 : Sum  Inputs=-|+  SaturateOnIntegerOverflow=on  InputSameDT=on  OutDataTypeStr=Inherit: Same as first input
  Sum12 : Sum  SaturateOnIntegerOverflow=on  InputSameDT=on  OutDataTypeStr=Inherit: Same as first input
  Sum6 : Sum  Inputs=-+|  SaturateOnIntegerOverflow=on  InputSameDT=on  OutDataTypeStr=Inherit: Same as first input
  Sum9 : Sum  Inputs=-+|  SaturateOnIntegerOverflow=on  InputSameDT=on  OutDataTypeStr=Inherit: Same as first input
  "abc --> dq " : Subsystem
  alpha2w2 : Integrator  InitialCondition=Isq_0_est2
  alpha2w4 : Integrator  InitialCondition=[Vsd_0; Vsq_0]
  "dq --> abc " : Subsystem
  w_mech_ref1 : Constant  Value=w_mech_rated
  Vs : Outport
  wires:
  Sum12/1 -> Demux3/1  "Vs_dq*"
  Demux1/2 -> "abc --> dq "/2(b)
  Demux1/1 -> "abc --> dq "/1(a)
  Demux1/3 -> "abc --> dq "/3(c)
  Is/1 -> Demux1/1
  "dq --> abc "/3(Vc) -> Mux5/3
  Sum6/1 -> Mux2/2
  "abc --> dq "/2(is_q) -> Sum6/1
  Demux3/1 -> "dq --> abc "/1(d)
  Sum10/1 -> Sum6/2  "isq*"
  Demux3/2 -> "dq --> abc "/2(q)
  Isd_ref/1 -> Sum9/2  "isd*"
  theta_da_est/1 -> "abc --> dq "/4(theta_da_est), "dq --> abc "/3(theta_da_est)
  alpha2w2/1 -> Sum10/1
  w_mech_ref1/1 -> Sum11/2
  w_mech1/1 -> Sum11/1
  "dq --> abc "/2(Vb) -> Mux5/2
  Gain2/1 -> alpha2w2/1
  "abc --> dq "/1(is_d) -> Sum9/1
  Mux5/1 -> Vs/1
  "dq --> abc "/1(Va) -> Mux5/1
  Mux2/1 -> Gain1/1, Gain8/1
  Gain1/1 -> alpha2w4/1
  Gain8/1 -> Sum12/2
  alpha2w4/1 -> Sum12/1
  Sum9/1 -> Mux2/1
  Gain7/1 -> Sum10/2
  Sum11/1 -> Gain2/1, Gain7/1

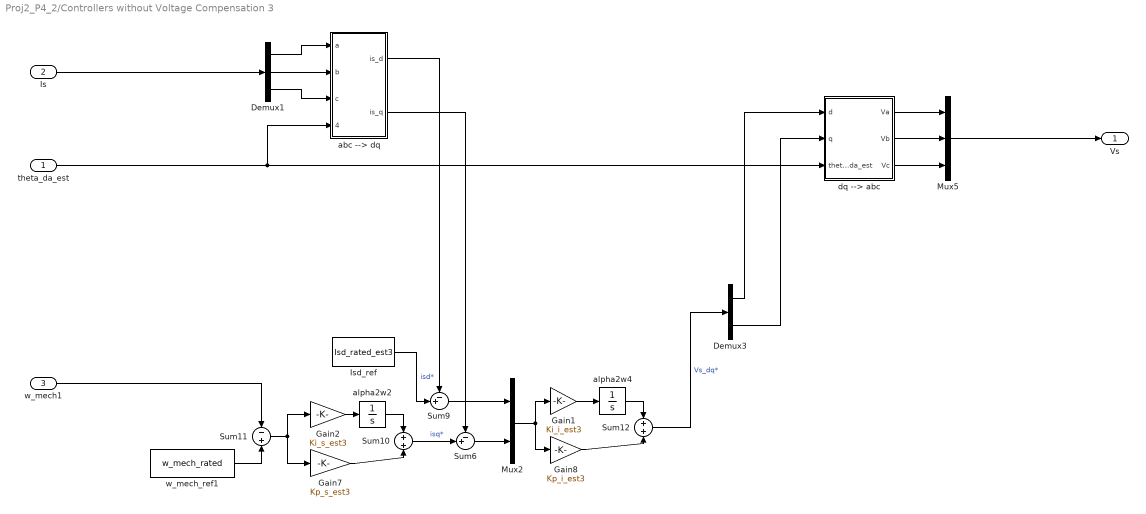
== system Proj2_P4_2/Controllers without Voltage Compensation 3 ==
  theta_da_est : Inport
  Is : Inport  Port=2
  w_mech1 : Inport  Port=3
  Demux1 : Demux  Outputs=3
  Demux3 : Demux  Outputs=2
  Gain1 : Gain  Gain=Ki_i_est3  SaturateOnIntegerOverflow=on  OutDataTypeStr=Inherit: Same as input  ParamDataTypeStr=Inherit: Same as input
  Gain2 : Gain  Gain=Ki_s_est3  SaturateOnIntegerOverflow=on  OutDataTypeStr=Inherit: Same as input  ParamDataTypeStr=Inherit: Same as input
  Gain7 : Gain  Gain=Kp_s_est3  SaturateOnIntegerOverflow=on  OutDataTypeStr=Inherit: Same as input  ParamDataTypeStr=Inherit: Same as input
  Gain8 : Gain  Gain=Kp_i_est3  SaturateOnIntegerOverflow=on  OutDataTypeStr=Inherit: Same as input  ParamDataTypeStr=Inherit: Same as input
  Isd_ref : Constant  Value=Isd_rated_est3
  Mux2 : Mux  Inputs=2
  Mux5 : Mux  Inputs=3
  Sum10 : Sum  SaturateOnIntegerOverflow=on  InputSameDT=on  OutDataTypeStr=Inherit: Same as first input
  Sum11 : Sum  Inputs=-|+  SaturateOnIntegerOverflow=on  InputSameDT=on  OutDataTypeStr=Inherit: Same as first input
  Sum12 : Sum  SaturateOnIntegerOverflow=on  InputSameDT=on  OutDataTypeStr=Inherit: Same as first input
  Sum6 : Sum  Inputs=-+|  SaturateOnIntegerOverflow=on  InputSameDT=on  OutDataTypeStr=Inherit: Same as first input
  Sum9 : Sum  Inputs=-+|  SaturateOnIntegerOverflow=on  InputSameDT=on  OutDataTypeStr=Inherit: Same as first input
  "abc --> dq " : Subsystem
  alpha2w2 : Integrator  InitialCondition=Isq_0_est3
  alpha2w4 : Integrator  InitialCondition=[Vsd_0; Vsq_0]
  "dq --> abc " : Subsystem
  w_mech_ref1 : Constant  Value=w_mech_rated
  Vs : Outport
  wires:
  Sum12/1 -> Demux3/1  "Vs_dq*"
  Demux1/2 -> "abc --> dq "/2(b)
  Demux1/1 -> "abc --> dq "/1(a)
  Demux1/3 -> "abc --> dq "/3(c)
  Is/1 -> Demux1/1
  "dq --> abc "/3(Vc) -> Mux5/3
  Sum6/1 -> Mux2/2
  "abc --> dq "/2(is_q) -> Sum6/1
  Demux3/1 -> "dq --> abc "/1(d)
  Sum10/1 -> Sum6/2  "isq*"
  Demux3/2 -> "dq --> abc "/2(q)
  Isd_ref/1 -> Sum9/2  "isd*"
  theta_da_est/1 -> "abc --> dq "/4(theta_da_est), "dq --> abc "/3(theta_da_est)
  alpha2w2/1 -> Sum10/1
  w_mech_ref1/1 -> Sum11/2
  w_mech1/1 -> Sum11/1
  "dq --> abc "/2(Vb) -> Mux5/2
  Gain2/1 -> alpha2w2/1
  "abc --> dq "/1(is_d) -> Sum9/1
  Mux5/1 -> Vs/1
  "dq --> abc "/1(Va) -> Mux5/1
  Mux2/1 -> Gain1/1, Gain8/1
  Gain1/1 -> alpha2w4/1
  Gain8/1 -> Sum12/2
  alpha2w4/1 -> Sum12/1
  Sum9/1 -> Mux2/1
  Gain7/1 -> Sum10/2
  Sum11/1 -> Gain2/1, Gain7/1

== system Proj2_P4_2/Double Click to load parameters and initial conditions  In this case, all initial values are obtained based on Actual Parameters;  parameters of Estimated Motor and Voltage Compensation Mode are based on Estimated Parameters;  paramters of  Controllers are based on Actual Parameters.   ==

== system Proj2_P4_2/Double Click to load parameters and initial conditions  In this case, all initial values are obtained based on Actual Parameters;  parameters of Estimated Motor and Voltage Compensation Model and Controllers are all based on Estimated Parameters   ==

== system Proj2_P4_2/Double Click to load parameters and initial conditions  In this case, all parameters and initial values in Estimated Motor, Voltage Compensation  and Controller Mode are based on Estimated Parameters ==

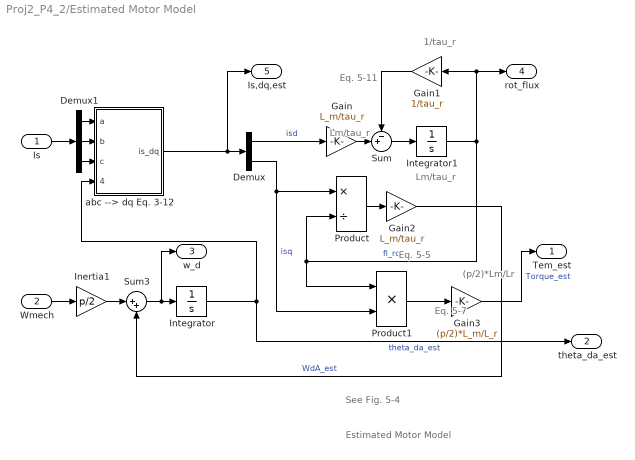
== system Proj2_P4_2/Estimated Motor Model ==
  note: See Fig. 5-4
  note: Eq. 5-7
  note: (p/2)*Lm/Lr
  note: Eq. 5-5
  note: Lm/tau_r
  note: Eq. 5-11
  note: 1/tau_r
  note: Lm/tau_r
  note: Estimated Motor Model
  Is : Inport
  Wmech : Inport  Port=2
  Demux : Demux  Outputs=2
  Demux1 : Demux  Outputs=3
  Gain : Gain  Gain=L_m/tau_r  SaturateOnIntegerOverflow=on  OutDataTypeStr=Inherit: Same as input  ParamDataTypeStr=Inherit: Same as input
  Gain1 : Gain  Gain=1/tau_r  SaturateOnIntegerOverflow=on  OutDataTypeStr=Inherit: Same as input  ParamDataTypeStr=Inherit: Same as input
  Gain2 : Gain  Gain=L_m/tau_r  SaturateOnIntegerOverflow=on  OutDataTypeStr=Inherit: Same as input  ParamDataTypeStr=Inherit: Same as input
  Gain3 : Gain  Gain=(p/2)*L_m/L_r  SaturateOnIntegerOverflow=on  OutDataTypeStr=Inherit: Same as input  ParamDataTypeStr=Inherit: Same as input
  Inertia1 : Gain  Gain=p/2  SaturateOnIntegerOverflow=on  OutDataTypeStr=Inherit: Same as input  ParamDataTypeStr=Inherit: Same as input
  Integrator : Integrator  InitialCondition=theta_da_0
  Integrator1 : Integrator  InitialCondition=fl_rd_0
  Product : Product  Inputs=*/  SaturateOnIntegerOverflow=on  RndMeth=Zero  InputSameDT=on  OutDataTypeStr=Inherit: Same as first input
  Product1 : Product  SaturateOnIntegerOverflow=on  RndMeth=Zero  InputSameDT=on  OutDataTypeStr=Inherit: Same as first input
  Sum : Sum  Inputs=-+|  SaturateOnIntegerOverflow=on  InputSameDT=on  OutDataTypeStr=Inherit: Same as first input
  Sum3 : Sum  Inputs=|++  SaturateOnIntegerOverflow=on  InputSameDT=on  OutDataTypeStr=Inherit: Same as first input
  abc --> dq Eq. 3-12 : Subsystem
  Tem_est : Outport
  theta_da_est : Outport  Port=2
  w_d : Outport  Port=3
  rot_flux : Outport  Port=4
  Is,dq,est : Outport  Port=5
  wires:
  Gain3/1 -> Tem_est/1  "Torque_est"
  Wmech/1 -> Inertia1/1
  Integrator/1 -> theta_da_est/1, abc --> dq Eq. 3-12/4(theta_da_est)  "theta_da_est"
  Gain2/1 -> Sum3/2  "WdA_est"
  Inertia1/1 -> Sum3/1
  Sum3/1 -> Integrator/1, w_d/1
  abc --> dq Eq. 3-12/1(is_dq) -> Is,dq,est/1, Demux/1
  Product1/1 -> Gain3/1
  Product/1 -> Gain2/1
  Demux/2 -> Product1/2, Product/1  "isq"
  Integrator1/1 -> Product1/1, Product/2, Gain1/1, rot_flux/1  "fl_rd"
  Sum/1 -> Integrator1/1
  Gain1/1 -> Sum/1
  Gain/1 -> Sum/2
  Demux/1 -> Gain/1  "isd"
  Demux1/1 -> abc --> dq Eq. 3-12/1(a)
  Demux1/2 -> abc --> dq Eq. 3-12/2(b)
  Demux1/3 -> abc --> dq Eq. 3-12/3(c)
  Is/1 -> Demux1/1

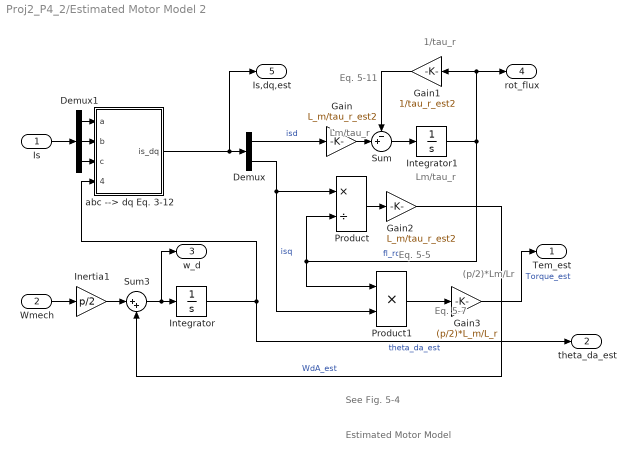
== system Proj2_P4_2/Estimated Motor Model 2 ==
  note: See Fig. 5-4
  note: Eq. 5-7
  note: (p/2)*Lm/Lr
  note: Eq. 5-5
  note: Lm/tau_r
  note: Eq. 5-11
  note: 1/tau_r
  note: Lm/tau_r
  note: Estimated Motor Model
  Is : Inport
  Wmech : Inport  Port=2
  Demux : Demux  Outputs=2
  Demux1 : Demux  Outputs=3
  Gain : Gain  Gain=L_m/tau_r_est2  SaturateOnIntegerOverflow=on  OutDataTypeStr=Inherit: Same as input  ParamDataTypeStr=Inherit: Same as input
  Gain1 : Gain  Gain=1/tau_r_est2  SaturateOnIntegerOverflow=on  OutDataTypeStr=Inherit: Same as input  ParamDataTypeStr=Inherit: Same as input
  Gain2 : Gain  Gain=L_m/tau_r_est2  SaturateOnIntegerOverflow=on  OutDataTypeStr=Inherit: Same as input  ParamDataTypeStr=Inherit: Same as input
  Gain3 : Gain  Gain=(p/2)*L_m/L_r  SaturateOnIntegerOverflow=on  OutDataTypeStr=Inherit: Same as input  ParamDataTypeStr=Inherit: Same as input
  Inertia1 : Gain  Gain=p/2  SaturateOnIntegerOverflow=on  OutDataTypeStr=Inherit: Same as input  ParamDataTypeStr=Inherit: Same as input
  Integrator : Integrator  InitialCondition=theta_da_0_est2
  Integrator1 : Integrator  InitialCondition=fl_rd_0_est2
  Product : Product  Inputs=*/  SaturateOnIntegerOverflow=on  RndMeth=Zero  InputSameDT=on  OutDataTypeStr=Inherit: Same as first input
  Product1 : Product  SaturateOnIntegerOverflow=on  RndMeth=Zero  InputSameDT=on  OutDataTypeStr=Inherit: Same as first input
  Sum : Sum  Inputs=-+|  SaturateOnIntegerOverflow=on  InputSameDT=on  OutDataTypeStr=Inherit: Same as first input
  Sum3 : Sum  Inputs=|++  SaturateOnIntegerOverflow=on  InputSameDT=on  OutDataTypeStr=Inherit: Same as first input
  abc --> dq Eq. 3-12 : Subsystem
  Tem_est : Outport
  theta_da_est : Outport  Port=2
  w_d : Outport  Port=3
  rot_flux : Outport  Port=4
  Is,dq,est : Outport  Port=5
  wires:
  Gain3/1 -> Tem_est/1  "Torque_est"
  Wmech/1 -> Inertia1/1
  Integrator/1 -> theta_da_est/1, abc --> dq Eq. 3-12/4(theta_da_est)  "theta_da_est"
  Gain2/1 -> Sum3/2  "WdA_est"
  Inertia1/1 -> Sum3/1
  Sum3/1 -> Integrator/1, w_d/1
  abc --> dq Eq. 3-12/1(is_dq) -> Is,dq,est/1, Demux/1
  Product1/1 -> Gain3/1
  Product/1 -> Gain2/1
  Demux/2 -> Product1/2, Product/1  "isq"
  Integrator1/1 -> Product1/1, Product/2, Gain1/1, rot_flux/1  "fl_rd"
  Sum/1 -> Integrator1/1
  Gain1/1 -> Sum/1
  Gain/1 -> Sum/2
  Demux/1 -> Gain/1  "isd"
  Demux1/1 -> abc --> dq Eq. 3-12/1(a)
  Demux1/2 -> abc --> dq Eq. 3-12/2(b)
  Demux1/3 -> abc --> dq Eq. 3-12/3(c)
  Is/1 -> Demux1/1

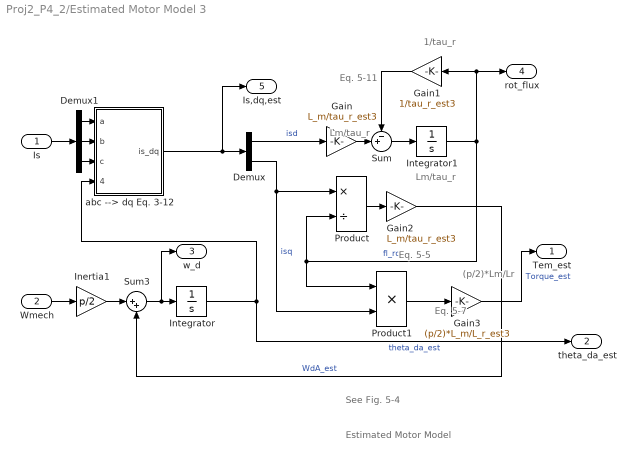
== system Proj2_P4_2/Estimated Motor Model 3 ==
  note: See Fig. 5-4
  note: Eq. 5-7
  note: (p/2)*Lm/Lr
  note: Eq. 5-5
  note: Lm/tau_r
  note: Eq. 5-11
  note: 1/tau_r
  note: Lm/tau_r
  note: Estimated Motor Model
  Is : Inport
  Wmech : Inport  Port=2
  Demux : Demux  Outputs=2
  Demux1 : Demux  Outputs=3
  Gain : Gain  Gain=L_m/tau_r_est3  SaturateOnIntegerOverflow=on  OutDataTypeStr=Inherit: Same as input  ParamDataTypeStr=Inherit: Same as input
  Gain1 : Gain  Gain=1/tau_r_est3  SaturateOnIntegerOverflow=on  OutDataTypeStr=Inherit: Same as input  ParamDataTypeStr=Inherit: Same as input
  Gain2 : Gain  Gain=L_m/tau_r_est3  SaturateOnIntegerOverflow=on  OutDataTypeStr=Inherit: Same as input  ParamDataTypeStr=Inherit: Same as input
  Gain3 : Gain  Gain=(p/2)*L_m/L_r_est3  SaturateOnIntegerOverflow=on  OutDataTypeStr=Inherit: Same as input  ParamDataTypeStr=Inherit: Same as input
  Inertia1 : Gain  Gain=p/2  SaturateOnIntegerOverflow=on  OutDataTypeStr=Inherit: Same as input  ParamDataTypeStr=Inherit: Same as input
  Integrator : Integrator  InitialCondition=theta_da_0_est3
  Integrator1 : Integrator  InitialCondition=fl_rd_0_est3
  Product : Product  Inputs=*/  SaturateOnIntegerOverflow=on  RndMeth=Zero  InputSameDT=on  OutDataTypeStr=Inherit: Same as first input
  Product1 : Product  SaturateOnIntegerOverflow=on  RndMeth=Zero  InputSameDT=on  OutDataTypeStr=Inherit: Same as first input
  Sum : Sum  Inputs=-+|  SaturateOnIntegerOverflow=on  InputSameDT=on  OutDataTypeStr=Inherit: Same as first input
  Sum3 : Sum  Inputs=|++  SaturateOnIntegerOverflow=on  InputSameDT=on  OutDataTypeStr=Inherit: Same as first input
  abc --> dq Eq. 3-12 : Subsystem
  Tem_est : Outport
  theta_da_est : Outport  Port=2
  w_d : Outport  Port=3
  rot_flux : Outport  Port=4
  Is,dq,est : Outport  Port=5
  wires:
  Gain3/1 -> Tem_est/1  "Torque_est"
  Wmech/1 -> Inertia1/1
  Integrator/1 -> theta_da_est/1, abc --> dq Eq. 3-12/4(theta_da_est)  "theta_da_est"
  Gain2/1 -> Sum3/2  "WdA_est"
  Inertia1/1 -> Sum3/1
  Sum3/1 -> Integrator/1, w_d/1
  abc --> dq Eq. 3-12/1(is_dq) -> Is,dq,est/1, Demux/1
  Product1/1 -> Gain3/1
  Product/1 -> Gain2/1
  Demux/2 -> Product1/2, Product/1  "isq"
  Integrator1/1 -> Product1/1, Product/2, Gain1/1, rot_flux/1  "fl_rd"
  Sum/1 -> Integrator1/1
  Gain1/1 -> Sum/1
  Gain/1 -> Sum/2
  Demux/1 -> Gain/1  "isd"
  Demux1/1 -> abc --> dq Eq. 3-12/1(a)
  Demux1/2 -> abc --> dq Eq. 3-12/2(b)
  Demux1/3 -> abc --> dq Eq. 3-12/3(c)
  Is/1 -> Demux1/1

== system Proj2_P4_2/Actual Motor dq Model Modified from EX5_3/abc --> dq Eq. 2.13 ==
  a : Inport
  b : Inport  Port=2
  c : Inport  Port=3
  theta_da : Inport  Port=4
  Mux1 : Mux
  Mux2 : Mux  Inputs=2
  vsd Eq. 3-12 : Fcn  Expr=sqrt(2/3)*(cos(u(4))*u(1)+cos(u(4)-2*pi/3)*u(2)+cos(u(4)-4*pi/3)*u(3))
  vsq Eq. 3-12 : Fcn  Expr=-sqrt(2/3)*(sin(u(4))*u(1)+sin(u(4)-2*pi/3)*u(2)+sin(u(4)-4*pi/3)*u(3))
  vs_dq : Outport
  wires:
  Mux1/1 -> vsd Eq. 3-12/1, vsq Eq. 3-12/1
  vsd Eq. 3-12/1 -> Mux2/1
  vsq Eq. 3-12/1 -> Mux2/2
  a/1 -> Mux1/1
  b/1 -> Mux1/2
  c/1 -> Mux1/3
  theta_da/1 -> Mux1/4
  Mux2/1 -> vs_dq/1

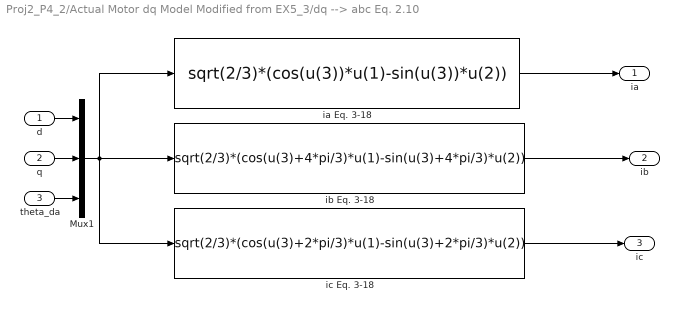
== system Proj2_P4_2/Actual Motor dq Model Modified from EX5_3/dq --> abc Eq. 2.10 ==
  d : Inport
  q : Inport  Port=2
  theta_da : Inport  Port=3
  Mux1 : Mux  Inputs=3
  ia Eq. 3-18 : Fcn  Expr=sqrt(2/3)*(cos(u(3))*u(1)-sin(u(3))*u(2))
  ib Eq. 3-18 : Fcn  Expr=sqrt(2/3)*(cos(u(3)+4*pi/3)*u(1)-sin(u(3)+4*pi/3)*u(2))
  ic Eq. 3-18 : Fcn  Expr=sqrt(2/3)*(cos(u(3)+2*pi/3)*u(1)-sin(u(3)+2*pi/3)*u(2))
  ia : Outport
  ib : Outport  Port=2
  ic : Outport  Port=3
  wires:
  ic Eq. 3-18/1 -> ic/1
  Mux1/1 -> ic Eq. 3-18/1, ib Eq. 3-18/1, ia Eq. 3-18/1
  ia Eq. 3-18/1 -> ia/1
  ib Eq. 3-18/1 -> ib/1
  d/1 -> Mux1/1
  q/1 -> Mux1/2
  theta_da/1 -> Mux1/3

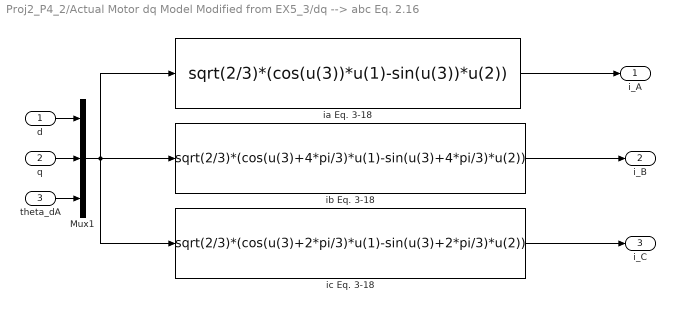
== system Proj2_P4_2/Actual Motor dq Model Modified from EX5_3/dq --> abc Eq. 2.16  ==
  d : Inport
  q : Inport  Port=2
  theta_dA : Inport  Port=3
  Mux1 : Mux  Inputs=3
  ia Eq. 3-18 : Fcn  Expr=sqrt(2/3)*(cos(u(3))*u(1)-sin(u(3))*u(2))
  ib Eq. 3-18 : Fcn  Expr=sqrt(2/3)*(cos(u(3)+4*pi/3)*u(1)-sin(u(3)+4*pi/3)*u(2))
  ic Eq. 3-18 : Fcn  Expr=sqrt(2/3)*(cos(u(3)+2*pi/3)*u(1)-sin(u(3)+2*pi/3)*u(2))
  i_A : Outport
  i_B : Outport  Port=2
  i_C : Outport  Port=3
  wires:
  ic Eq. 3-18/1 -> i_C/1
  Mux1/1 -> ic Eq. 3-18/1, ib Eq. 3-18/1, ia Eq. 3-18/1
  ib Eq. 3-18/1 -> i_B/1
  d/1 -> Mux1/1
  q/1 -> Mux1/2
  theta_dA/1 -> Mux1/3
  ia Eq. 3-18/1 -> i_A/1

== system Proj2_P4_2/Actual Motor dq Model Modified from EX5_3/stator_flux Eq. 2.28 ==
  vs_dq : Inport
  is_dq : Inport  Port=2
  w_d : Inport  Port=3
  Gain : Gain  Gain=R_s  SaturateOnIntegerOverflow=on  OutDataTypeStr=Inherit: Same as input  ParamDataTypeStr=Inherit: Same as input
  Integrator1 : Integrator  InitialCondition=[fl_sd_0; fl_sq_0]
  "Matrix [0 -1  1 0] " : Gain  Gain=[0 -1; 1 0]  Multiplication=Matrix(K*u)  SaturateOnIntegerOverflow=on  OutDataTypeStr=Inherit: Same as input  ParamDataTypeStr=Inherit: Same as input
  Product : Product  SaturateOnIntegerOverflow=on  RndMeth=Zero  InputSameDT=on  OutDataTypeStr=Inherit: Same as first input
  Sum : Sum  Inputs=-+-  SaturateOnIntegerOverflow=on  InputSameDT=on  OutDataTypeStr=Inherit: Same as first input
  fl_s_dq : Outport
  wires:
  Sum/1 -> Integrator1/1
  Integrator1/1 -> "Matrix [0 -1  1 0] "/1, fl_s_dq/1
  "Matrix [0 -1  1 0] "/1 -> Product/2
  Product/1 -> Sum/1
  w_d/1 -> Product/1
  vs_dq/1 -> Sum/2
  is_dq/1 -> Gain/1
  Gain/1 -> Sum/3

== system Proj2_P4_2/Actual Motor dq Model Modified from EX5_3 /abc --> dq Eq. 2.13 ==
  a : Inport
  b : Inport  Port=2
  c : Inport  Port=3
  theta_da : Inport  Port=4
  Mux1 : Mux
  Mux2 : Mux  Inputs=2
  vsd Eq. 3-12 : Fcn  Expr=sqrt(2/3)*(cos(u(4))*u(1)+cos(u(4)-2*pi/3)*u(2)+cos(u(4)-4*pi/3)*u(3))
  vsq Eq. 3-12 : Fcn  Expr=-sqrt(2/3)*(sin(u(4))*u(1)+sin(u(4)-2*pi/3)*u(2)+sin(u(4)-4*pi/3)*u(3))
  vs_dq : Outport
  wires:
  Mux1/1 -> vsd Eq. 3-12/1, vsq Eq. 3-12/1
  vsd Eq. 3-12/1 -> Mux2/1
  vsq Eq. 3-12/1 -> Mux2/2
  a/1 -> Mux1/1
  b/1 -> Mux1/2
  c/1 -> Mux1/3
  theta_da/1 -> Mux1/4
  Mux2/1 -> vs_dq/1

== system Proj2_P4_2/Actual Motor dq Model Modified from EX5_3 /dq --> abc Eq. 2.10 ==
  d : Inport
  q : Inport  Port=2
  theta_da : Inport  Port=3
  Mux1 : Mux  Inputs=3
  ia Eq. 3-18 : Fcn  Expr=sqrt(2/3)*(cos(u(3))*u(1)-sin(u(3))*u(2))
  ib Eq. 3-18 : Fcn  Expr=sqrt(2/3)*(cos(u(3)+4*pi/3)*u(1)-sin(u(3)+4*pi/3)*u(2))
  ic Eq. 3-18 : Fcn  Expr=sqrt(2/3)*(cos(u(3)+2*pi/3)*u(1)-sin(u(3)+2*pi/3)*u(2))
  ia : Outport
  ib : Outport  Port=2
  ic : Outport  Port=3
  wires:
  ic Eq. 3-18/1 -> ic/1
  Mux1/1 -> ic Eq. 3-18/1, ib Eq. 3-18/1, ia Eq. 3-18/1
  ia Eq. 3-18/1 -> ia/1
  ib Eq. 3-18/1 -> ib/1
  d/1 -> Mux1/1
  q/1 -> Mux1/2
  theta_da/1 -> Mux1/3

== system Proj2_P4_2/Actual Motor dq Model Modified from EX5_3 /dq --> abc Eq. 2.16  ==
  d : Inport
  q : Inport  Port=2
  theta_dA : Inport  Port=3
  Mux1 : Mux  Inputs=3
  ia Eq. 3-18 : Fcn  Expr=sqrt(2/3)*(cos(u(3))*u(1)-sin(u(3))*u(2))
  ib Eq. 3-18 : Fcn  Expr=sqrt(2/3)*(cos(u(3)+4*pi/3)*u(1)-sin(u(3)+4*pi/3)*u(2))
  ic Eq. 3-18 : Fcn  Expr=sqrt(2/3)*(cos(u(3)+2*pi/3)*u(1)-sin(u(3)+2*pi/3)*u(2))
  i_A : Outport
  i_B : Outport  Port=2
  i_C : Outport  Port=3
  wires:
  ic Eq. 3-18/1 -> i_C/1
  Mux1/1 -> ic Eq. 3-18/1, ib Eq. 3-18/1, ia Eq. 3-18/1
  ib Eq. 3-18/1 -> i_B/1
  d/1 -> Mux1/1
  q/1 -> Mux1/2
  theta_dA/1 -> Mux1/3
  ia Eq. 3-18/1 -> i_A/1

== system Proj2_P4_2/Actual Motor dq Model Modified from EX5_3 /stator_flux Eq. 2.28 ==
  vs_dq : Inport
  is_dq : Inport  Port=2
  w_d : Inport  Port=3
  Gain : Gain  Gain=R_s  SaturateOnIntegerOverflow=on  OutDataTypeStr=Inherit: Same as input  ParamDataTypeStr=Inherit: Same as input
  Integrator1 : Integrator  InitialCondition=[fl_sd_0; fl_sq_0]
  "Matrix [0 -1  1 0] " : Gain  Gain=[0 -1; 1 0]  Multiplication=Matrix(K*u)  SaturateOnIntegerOverflow=on  OutDataTypeStr=Inherit: Same as input  ParamDataTypeStr=Inherit: Same as input
  Product : Product  SaturateOnIntegerOverflow=on  RndMeth=Zero  InputSameDT=on  OutDataTypeStr=Inherit: Same as first input
  Sum : Sum  Inputs=-+-  SaturateOnIntegerOverflow=on  InputSameDT=on  OutDataTypeStr=Inherit: Same as first input
  fl_s_dq : Outport
  wires:
  Sum/1 -> Integrator1/1
  Integrator1/1 -> "Matrix [0 -1  1 0] "/1, fl_s_dq/1
  "Matrix [0 -1  1 0] "/1 -> Product/2
  Product/1 -> Sum/1
  w_d/1 -> Product/1
  vs_dq/1 -> Sum/2
  is_dq/1 -> Gain/1
  Gain/1 -> Sum/3

== system Proj2_P4_2/Actual Motor dq Model Modified from EX5_3  /abc --> dq Eq. 2.13 ==
  a : Inport
  b : Inport  Port=2
  c : Inport  Port=3
  theta_da : Inport  Port=4
  Mux1 : Mux
  Mux2 : Mux  Inputs=2
  vsd Eq. 3-12 : Fcn  Expr=sqrt(2/3)*(cos(u(4))*u(1)+cos(u(4)-2*pi/3)*u(2)+cos(u(4)-4*pi/3)*u(3))
  vsq Eq. 3-12 : Fcn  Expr=-sqrt(2/3)*(sin(u(4))*u(1)+sin(u(4)-2*pi/3)*u(2)+sin(u(4)-4*pi/3)*u(3))
  vs_dq : Outport
  wires:
  Mux1/1 -> vsd Eq. 3-12/1, vsq Eq. 3-12/1
  vsd Eq. 3-12/1 -> Mux2/1
  vsq Eq. 3-12/1 -> Mux2/2
  a/1 -> Mux1/1
  b/1 -> Mux1/2
  c/1 -> Mux1/3
  theta_da/1 -> Mux1/4
  Mux2/1 -> vs_dq/1

== system Proj2_P4_2/Actual Motor dq Model Modified from EX5_3  /dq --> abc Eq. 2.10 ==
  d : Inport
  q : Inport  Port=2
  theta_da : Inport  Port=3
  Mux1 : Mux  Inputs=3
  ia Eq. 3-18 : Fcn  Expr=sqrt(2/3)*(cos(u(3))*u(1)-sin(u(3))*u(2))
  ib Eq. 3-18 : Fcn  Expr=sqrt(2/3)*(cos(u(3)+4*pi/3)*u(1)-sin(u(3)+4*pi/3)*u(2))
  ic Eq. 3-18 : Fcn  Expr=sqrt(2/3)*(cos(u(3)+2*pi/3)*u(1)-sin(u(3)+2*pi/3)*u(2))
  ia : Outport
  ib : Outport  Port=2
  ic : Outport  Port=3
  wires:
  ic Eq. 3-18/1 -> ic/1
  Mux1/1 -> ic Eq. 3-18/1, ib Eq. 3-18/1, ia Eq. 3-18/1
  ia Eq. 3-18/1 -> ia/1
  ib Eq. 3-18/1 -> ib/1
  d/1 -> Mux1/1
  q/1 -> Mux1/2
  theta_da/1 -> Mux1/3

== system Proj2_P4_2/Actual Motor dq Model Modified from EX5_3  /dq --> abc Eq. 2.16  ==
  d : Inport
  q : Inport  Port=2
  theta_dA : Inport  Port=3
  Mux1 : Mux  Inputs=3
  ia Eq. 3-18 : Fcn  Expr=sqrt(2/3)*(cos(u(3))*u(1)-sin(u(3))*u(2))
  ib Eq. 3-18 : Fcn  Expr=sqrt(2/3)*(cos(u(3)+4*pi/3)*u(1)-sin(u(3)+4*pi/3)*u(2))
  ic Eq. 3-18 : Fcn  Expr=sqrt(2/3)*(cos(u(3)+2*pi/3)*u(1)-sin(u(3)+2*pi/3)*u(2))
  i_A : Outport
  i_B : Outport  Port=2
  i_C : Outport  Port=3
  wires:
  ic Eq. 3-18/1 -> i_C/1
  Mux1/1 -> ic Eq. 3-18/1, ib Eq. 3-18/1, ia Eq. 3-18/1
  ib Eq. 3-18/1 -> i_B/1
  d/1 -> Mux1/1
  q/1 -> Mux1/2
  theta_dA/1 -> Mux1/3
  ia Eq. 3-18/1 -> i_A/1

== system Proj2_P4_2/Actual Motor dq Model Modified from EX5_3  /stator_flux Eq. 2.28 ==
  vs_dq : Inport
  is_dq : Inport  Port=2
  w_d : Inport  Port=3
  Gain : Gain  Gain=R_s  SaturateOnIntegerOverflow=on  OutDataTypeStr=Inherit: Same as input  ParamDataTypeStr=Inherit: Same as input
  Integrator1 : Integrator  InitialCondition=[fl_sd_0; fl_sq_0]
  "Matrix [0 -1  1 0] " : Gain  Gain=[0 -1; 1 0]  Multiplication=Matrix(K*u)  SaturateOnIntegerOverflow=on  OutDataTypeStr=Inherit: Same as input  ParamDataTypeStr=Inherit: Same as input
  Product : Product  SaturateOnIntegerOverflow=on  RndMeth=Zero  InputSameDT=on  OutDataTypeStr=Inherit: Same as first input
  Sum : Sum  Inputs=-+-  SaturateOnIntegerOverflow=on  InputSameDT=on  OutDataTypeStr=Inherit: Same as first input
  fl_s_dq : Outport
  wires:
  Sum/1 -> Integrator1/1
  Integrator1/1 -> "Matrix [0 -1  1 0] "/1, fl_s_dq/1
  "Matrix [0 -1  1 0] "/1 -> Product/2
  Product/1 -> Sum/1
  w_d/1 -> Product/1
  vs_dq/1 -> Sum/2
  is_dq/1 -> Gain/1
  Gain/1 -> Sum/3
